simulink model "Revised_model_charging_station"  (Simulink 10.3)
settings: Solver=ode8  StartTime=0.0  StopTime=6  FixedStep=1e-04  RelTol=1e-3
undefined symbols (not defined in the file or in its folder): Acid, Lead
libraries: spsMosfetLib x14, spsDiodeLib x13, spsSeriesRLCBranchLib x12, simulink x9, spsCurrentMeasurementLib x8, pid_lib x7, spsBatteryLib x6, spsParallelRLCBranchLib x5, spsMeanLib x3, spsGroundLib x2, spsPWMGeneratorDCDCLib x2, spsVoltageMeasurementLib x2
settings Model: Creator=Devershi  LastModifiedBy=Aditya
settings Model: SuppressorTable=|
  | <?xml version="1.0" encoding="UTF-8" standalone="yes" ?>
  | <!DOCTYPE boost_serialization>
  | <boost_serialization signature="serialization::archive" version="17">
  | <DiagnosticSuppressor class_id="0" tracking_level="0" version="7">
  | 	<Table class_id="1" tracking_level="0" version="0">
  | 		<count>1</count>
  | 		<bucket_count>8</bucket_count>
  | 		<item_version>0</item_version>
  | 		<item class_id="2" tracking_level="0" version="0">
  | 			<first class_id="3" tracking_level="0" version="7">
  | 				<Source class_id="4" tracking_level="0" version="0">
  | 					<count>1</count>
  | 					<item_version>0</item_version>
  | 					<item>84:4</item>
  | 				</Source>
  | 			</first>
  | 			<second class_id="5" tracking_level="0" version="7">
  | 				<SuppressedData class_id="6" tracking_level="0" version="0">
  | 					<count>2</count>
  | 					<bucket_count>8</bucket_count>
  | 					<item_version>0</item_version>
  | 					<item class_id="7" tracking_level="0" version="0">
  | 						<first class_id="8" tracking_level="0" version="7">
  | 							<ID>SimulinkFixedPoint:util:Overflowoccurred</ID>
  | 							<Cause>
  | 								<Source>
  | 									<count>0</count>
  | 									<item_version>0</item_version>
  | 								</Source>
  | 							</Cause>
  | 						</first>
  | 						<second class_id="9" tracking_level="0" version="7">
  | 							<Comment></Comment>
  | 							<User></User>
  | 							<LastModified class_id="10" tracking_level="0" version="0">
  | 								<ptime_date class_id="11" tracking_level="0" version="0">
  | 									<date>20160608</date>
  | 								</ptime_date>
  | 								<ptime_time_duration class_id="12" tracking_level="0" version="1">
  | 									<is_special>0</is_special>
  | 									<time_duration_hours>15</time_duration_hours>
  | 									<time_duration_minutes>23</time_duration_minutes>
  | 									<time_duration_seconds>17</time_duration_seconds>
  | 									<time_duration_fractional_seconds>0</time_duration_fractional_seconds>
  | 								</ptime_time_duration>
  | 							</LastModified>
  | 							<SuppressionType>1</SuppressionType>
  | 						</second>
  | 					</item>
  | 					<item>
  | 						<first>
  | 							<ID>Simulink:DataType:WarningOverFlowDetected</ID>
  | 							<Cause>
  | 								<Source>
  | 									<count>0</count>
  | 									<item_version>0</item_version>
  | 								</Source>
  | 							</Cause>
  | 						</first>
  | 						<second>
  | 							<Comment></Comment>
  | 							<User></User>
  | 							<LastModified>
  | 								<ptime_date>
  | 									<date>20160608</date>
  | 								</ptime_date>
  | 								<ptime_time_duration>
  | 									<is_special>0</is_special>
  | 									<time_duration_hours>15</time_duration_hours>
  | 									<time_duration_minutes>23</time_duration_minutes>
  | 									<time_duration_seconds>17</time_duration_seconds>
  | 									<time_duration_fractional_seconds>0</time_duration_fractional_seconds>
  | 								</ptime_time_duration>
  | 							</LastModified>
  | 							<SuppressionType>1</SuppressionType>
  | 						</second>
  | 					</item>
  | 				</SuppressedData>
  | 			</second>
  | 		</item>
  | 	</Table>
  | </DiagnosticSuppressor>
  | 
  | </boost_serialization>
  | 
  | </boost_serialization>
settings SolverCC: AlgebraicLoopSolver=Auto
settings DataIOCC: SaveFormat=Dataset  SignalLoggingSaveFormat=Dataset  ReturnWorkspaceOutputs=on
settings OptimizationCC: ExpressionDepthLimit=128  LifeSpan=auto
settings DebuggingCC: UnderspecifiedInitializationDetection=Simplified  MergeDetectMultiDrivingBlocksExec=error  FcnCallInpInsideContextMsg=error  StateNameClashWarn=none  SFUnexpectedBacktrackingDiag=error  SFNoUnconditionalDefaultTransitionDiag=error  SFExecutionAtInitializationDiag=warning  SFMachineParentedDataDiag=error  ArithmeticOperatorsInVariantConditions=error
settings HardwareCC: ProdBitPerPointer=64  ProdBitPerSizeT=64  ProdBitPerPtrDiffT=64  ProdLargestAtomicFloat=Float  ProdIntDivRoundTo=Zero  ProdEndianess=LittleEndian  ProdWordSize=64  ProdHWDeviceType=Intel->x86-64 (Windows64)
settings ModelReferenceCC: PropagateSignalLabelsOutOfModel=on
settings SFSimCC: SimUseLocalCustomCode=on  CustomCodeUndefinedFunction=FilterOut
settings RTWCC: RTWUseLocalCustomCode=on
settings CodeAppCC: StateflowObjectComments=off
settings GRTTargetCC: TargetLangStandard=C99 (ISO)  CombineOutputUpdateFcns=on  GRTInterface=off
settings ConfigComp: CovMetricSettings=dwe  CovSaveCumulativeToWorkspaceVar=off  CovSaveSingleToWorkspaceVar=off  CovExternalEMLEnable=on

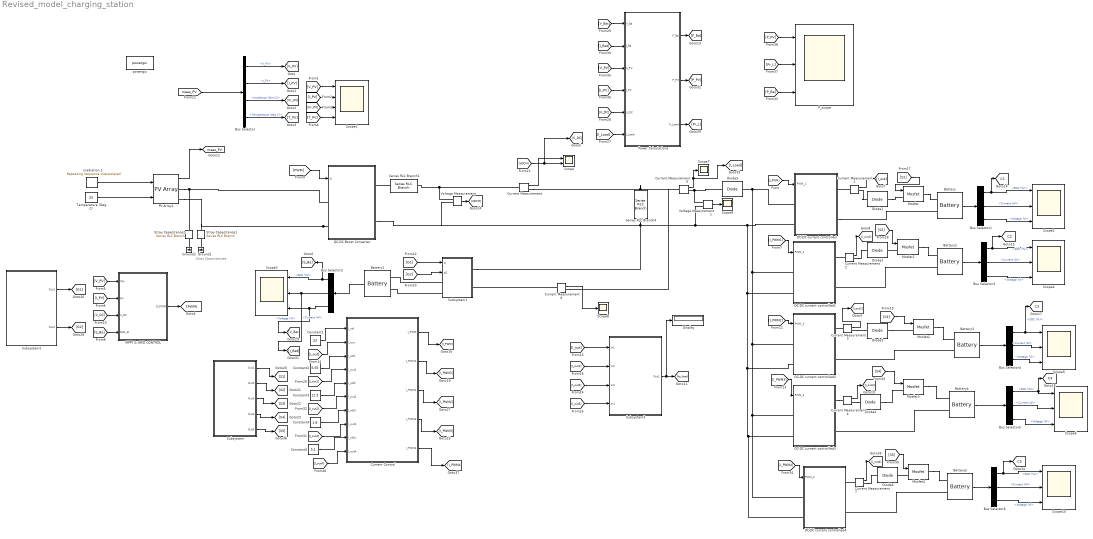
== system Revised_model_charging_station ==
  note: Stray
      | Capacitances
  Battery : spsBatteryLib/Battery  BatType=Lead-Acid  ShowTempParam=off  ThermalPreset=no  ShowAgeParam=off  NomV=72  NomQ=100  SOC=60  Batt_Tr=0.1  PresetModel=on  MaxQ=104.1667  MinV=54  FullV=78.3947  Dis_rate=20  R=0.0072  Normal_OP=31.0278  expZone="[73.3026     0.333333]"  current=[6.5 13 32.5]  Units=Time  Tci=20  NomT=20  T2=-30  MaxQ2=4.8  FullV2=7.1  Normal_OP2=5.655  expZone2="[6.58           1]"  Rca=0.6  ti=2000  Dp=0  Neq0=0  Tsim=1e6  Ta1=25  Qeol=5.4*0.9  Reol=0.013333*1.2  Char_age=[2.3478, 3]  Dis_age=[2.3478, 10]  N1=1500  N2=10500  N3=1000  N4=1400  Ta2=45  N5=950
  Battery1 : spsBatteryLib/Battery  BatType=Lead-Acid  ShowTempParam=off  ThermalPreset=no  ShowAgeParam=off  NomV=100  NomQ=150  SOC=65  Batt_Tr=0.1  PresetModel=on  MaxQ=156.25  MinV=75  FullV=108.8816  Dis_rate=30  R=0.0066667  Normal_OP=46.5417  expZone="[101.8092           0.5]"  current=[6.5 13 32.5]  Units=Time  Tci=20  NomT=20  T2=-30  MaxQ2=4.8  FullV2=7.1  Normal_OP2=5.655  expZone2="[6.58           1]"  Rca=0.6  ti=2000  Dp=0  Neq0=0  Tsim=1e6  Ta1=25  Qeol=5.4*0.9  Reol=0.013333*1.2  Char_age=[2.3478, 3]  Dis_age=[2.3478, 10]  N1=1500  N2=10500  N3=1000  N4=1400  Ta2=45  N5=950
  Battery2 : spsBatteryLib/Battery  BatType=Lead-Acid  ShowTempParam=off  ThermalPreset=no  ShowAgeParam=off  NomV=48  NomQ=37  SOC=30  Batt_Tr=0.1  PresetModel=on  MaxQ=38.5417  MinV=36  FullV=52.2632  Dis_rate=7.4  R=0.012973  Normal_OP=11.4803  expZone="[48.8684     0.123333]"  current=[6.5 13 32.5]  Units=Time  Tci=20  NomT=20  T2=-30  MaxQ2=4.8  FullV2=7.1  Normal_OP2=5.655  expZone2="[6.58           1]"  Rca=0.6  ti=2000  Dp=0  Neq0=0  Tsim=1e6  Ta1=25  Qeol=5.4*0.9  Reol=0.013333*1.2  Char_age=[2.3478, 3]  Dis_age=[2.3478, 10]  N1=1500  N2=10500  N3=1000  N4=1400  Ta2=45  N5=950
  Battery3 : spsBatteryLib/Battery  BatType=Lead-Acid  ShowTempParam=off  ThermalPreset=no  ShowAgeParam=off  NomV=48  NomQ=50  SOC=15  Batt_Tr=0.1  PresetModel=on  MaxQ=52.0833  MinV=36  FullV=52.2632  Dis_rate=10  R=0.0096  Normal_OP=15.5139  expZone="[48.8684     0.166667]"  current=[6.5 13 32.5]  Units=Time  Tci=20  NomT=20  T2=-30  MaxQ2=4.8  FullV2=7.1  Normal_OP2=5.655  expZone2="[6.58           1]"  Rca=0.6  ti=2000  Dp=0  Neq0=0  Tsim=1e6  Ta1=25  Qeol=5.4*0.9  Reol=0.013333*1.2  Char_age=[2.3478, 3]  Dis_age=[2.3478, 10]  N1=1500  N2=10500  N3=1000  N4=1400  Ta2=45  N5=950
  Battery4 : spsBatteryLib/Battery  BatType=Lead-Acid  ShowTempParam=off  ThermalPreset=no  ShowAgeParam=off  NomV=12  NomQ=18  SOC=90  Batt_Tr=0.1  PresetModel=on  MaxQ=18.75  MinV=9  FullV=13.0658  Dis_rate=3.6  R=0.0066667  Normal_OP=5.585  expZone="[12.2171         0.06]"  current=[6.5 13 32.5]  Units=Time  Tci=20  NomT=20  T2=-30  MaxQ2=4.8  FullV2=7.1  Normal_OP2=5.655  expZone2="[6.58           1]"  Rca=0.6  ti=2000  Dp=0  Neq0=0  Tsim=1e6  Ta1=25  Qeol=5.4*0.9  Reol=0.013333*1.2  Char_age=[2.3478, 3]  Dis_age=[2.3478, 10]  N1=1500  N2=10500  N3=1000  N4=1400  Ta2=45  N5=950
  Battery5 : spsBatteryLib/Battery  BatType=Lead-Acid  ShowTempParam=off  ThermalPreset=no  ShowAgeParam=off  NomV=48  NomQ=34  SOC=72  Batt_Tr=0.1  PresetModel=on  MaxQ=35.4167  MinV=36  FullV=52.2632  Dis_rate=6.8  R=0.014118  Normal_OP=10.5494  expZone="[48.8684     0.113333]"  current=[6.5 13 32.5]  Units=Time  Tci=20  NomT=20  T2=-30  MaxQ2=4.8  FullV2=7.1  Normal_OP2=5.655  expZone2="[6.58           1]"  Rca=0.6  ti=2000  Dp=0  Neq0=0  Tsim=1e6  Ta1=25  Qeol=5.4*0.9  Reol=0.013333*1.2  Char_age=[2.3478, 3]  Dis_age=[2.3478, 10]  N1=1500  N2=10500  N3=1000  N4=1400  Ta2=45  N5=950
  Bus Selector : BusSelector  OutputSignals=V_PV,I_PV,Irradiance (W/m2),Temperature (deg C)
  Bus Selector{1..6} (6 alike) : BusSelector  OutputSignals=SOC (%),Current (A),Voltage (V)
  Constant1 : Constant  Value=23
  Constant2 : Constant  Value=5.55
  Constant3 : Constant  Value=11.5
  Constant4 : Constant  Value=1.8
  Constant5 : Constant  Value=5.1
  Current Control : Subsystem
  Current Measurement{,1..7} (8 alike) : spsCurrentMeasurementLib/Current Measurement  PhasorSimulation=off  OutputType=Complex  PSBequivalent=0
  DC-DC Boost Converter : Subsystem
  DC-DC current controlled : Subsystem
  DC-DC current controlled1 : Subsystem
  DC-DC current controlled2 : Subsystem
  DC-DC current controlled3 : Subsystem
  DC-DC current controlled4 : Subsystem
  Diode{1..6} (6 alike) : spsDiodeLib/Diode  Ron=0.001  Lon=0  Vf=0.8  IC=0  UseSnubber=0  Rs=500  Cs=250e-9  Measurements=off
  Display : Display
  Ground1 : spsGroundLib/Ground  LConnTagsString=a
  Ground2 : spsGroundLib/Ground  LConnTagsString=a
  MPPT & GRID CONTROL : Subsystem
  Mosfet{,1..4} (5 alike) : spsMosfetLib/Mosfet  Ron=0.1  Lon=0  Rd=0.01  Vfd=0  IC=0  Rs=1e5  Cs=inf  Measurements=off
  PV Array1 : spsPVArrayLib/PV Array  Npar=8  Nser=8  PlotType=one module @ 25 deg.C & specified irradiances  S_vec="[ 1000 800 500  250 ]"  Temp_C_vec="[0 25 50  ]"  ModuleName=User-defined  PlotWhenSelected=on  Pm=204.7968  Ncell=60  Voc=22.46  Isc=11.65  Vm=18.72  Im=10.94  beta_Voc_pc=-0.3609  alpha_Isc_pc=0.102  beta_Voc=-0.081058  alpha_Isc=0.011883  IL=11.6575  I0=4.2837e-10  nI=0.60677  Rsh=131.4101  Rs=0.084786  RobustModel=off  RobustCellTemperature=25  BAL=on  Tc=Tc  Tfilter=5e-5
  P_scope : Scope  NumInputPorts=3
  Power Calculations : Subsystem
  Scope : Scope  NumInputPorts=2
  Scope1 : Scope  NumInputPorts=4
  Scope{2..6,10} (6 alike) : Scope  NumInputPorts=3
  Scope7 : Scope
  Scope8 : Scope
  Scope9 : Scope
  Series RLC Branch1 : spsSeriesRLCBranchLib/Series RLC Branch  LConnTagsString=__new0  RConnTagsString=__new0  BranchType=L  Resistance=1  Inductance=0.325e-3  SetiL0=off  InitialCurrent=0  Capacitance=15000e-6  Setx0=on  InitialVoltage=70  Measurements=None
  Series RLC Branch4 : spsSeriesRLCBranchLib/Series RLC Branch  LConnTagsString=__new0  RConnTagsString=__new0  BranchType=C  Resistance=1  Inductance=1e-3  SetiL0=off  InitialCurrent=0  Capacitance=15000e-6  Setx0=on  InitialVoltage=60  Measurements=None
  Stray Capacitance1 : spsSeriesRLCBranchLib/Series RLC Branch  LConnTagsString=__new0  RConnTagsString=__new0  BranchType=C  Resistance=1e-3  Inductance=1  SetiL0=off  InitialCurrent=0  Capacitance=4e-9  Setx0=off  InitialVoltage=0  Measurements=None
  Stray Capacitance2 : spsSeriesRLCBranchLib/Series RLC Branch  LConnTagsString=__new0  RConnTagsString=__new0  BranchType=C  Resistance=1e-3  Inductance=1  SetiL0=off  InitialCurrent=0  Capacitance=4e-9  Setx0=off  InitialVoltage=0  Measurements=None
  Subsystem : Subsystem
  Subsystem1 : Subsystem
  Subsystem2 : Subsystem
  Subsystem3 : Subsystem
  Temperature (Deg. C) : Constant  Value=25
  Voltage Measurement : spsVoltageMeasurementLib/Voltage Measurement  PhasorSimulation=off  OutputType=Complex  PSBequivalent=0
  Voltage Measurement1 : spsVoltageMeasurementLib/Voltage Measurement  PhasorSimulation=off  OutputType=Complex  PSBequivalent=0
  irradiation 2 : simulink/Sources/Repeating Sequence Interpolated  OutValues="[0 0  0 0 0 100 200 300 400 700 800 900 1000 975 900 800 700 400 300 200 0 0 0 0  ].'"  TimeValues=[0 0.25 0.50 0.75 1 1.25 1.50 1.75 2 2.25 2.75 3 3.25 3.50 3.75 4 4.25 4.5 4.75 5 5.25 5.5 5.75 6 ].'  LookUpMeth=Interpolation-Use End Values  tsamp=0.1  OutMin=[]  OutMax=[]  OutDataTypeStr=double  OutputDataTypeScalingMode=double  OutDataType=fixdt(0,8)  OutScaling=2^-10
  powergui : spspowerguiLib/powergui  Priority=1  SimulationMode=Discrete  SampleTime=1e-4  frequency=60  Iterations=50  frequencyindice=0  Pbase=100e6  ErrMax=1e-4  UnitsV=kV  UnitsW=MW  buscounter=0  FunctionMessages=off  echomessages=off  EnableUseOfTLC=off  CurrentSourceSwitches=off  DisableSnubberDevices=off  DisableRonSwitches=off  DisableVfSwitches=off  DisplayEquations=off  AutomaticDiscreteSolvers=off  SolverType=Tustin/Backward Euler (TBE)  Interpol=off  ExternalGateDelay=off  methode=off  Ts=100  x0status=blocks  SPID=on  SwTol=0  HookPort=off  NonlinearTolerance=1e-4  nMaxIteration=100  ContinueOnMaxIteration=off  RestoreLinks=warning  ResistiveCurrentMeasurement=off  Frange=[0:2:500]  Ylog=off  Xlog=on  ShowGrid=off  save=off  variable=ZData  structure=V_BATT  ZoomFFT=on  StartTime=0.604  cycles=7  DisplayStyle=1  fundamental=50  FreqAxis=off  MaxFrequency=200  frequencyindicesteady=1  RmsSteady=1  display=off
  tag scope: C1=global, C2=global, C3=global, C4=global, C5=global, No_load=global, meas_PV=global
  wires:
  Bus Selector5/2 -> Scope6/2  "<Current (A)>"
  Bus Selector5/3 -> Scope6/3  "<Voltage (V)>"
  Bus Selector5/1 -> [C4], Scope6/1  "<SOC (%)>"
  Battery2/1 -> Bus Selector3/1
  Bus Selector3/3 -> Scope4/3  "<Voltage (V)>"
  Bus Selector3/2 -> Scope4/2  "<Current (A)>"
  Battery/1 -> Bus Selector1/1
  Bus Selector1/3 -> Scope2/3  "<Voltage (V)>"
  Bus Selector/4 -> [T_PV]  "<Temperature (deg C)>"
  [meas_PV] -> Bus Selector/1
  [T_PV] -> Scope1/4
  Bus Selector/3 -> [Irr_PV]  "<Irradiance (W/m2)>"
  [I_PV] -> Scope1/2
  Bus Selector4/2 -> Scope5/2  "<Current (A)>"
  Bus Selector4/1 -> [C3], Scope5/1  "<SOC (%)>"
  Bus Selector/1 -> [V_PV]  "<V_PV>"
  Battery4/1 -> Bus Selector5/1
  Bus Selector/2 -> [I_PV]  "<I_PV>"
  [Irr_PV] -> Scope1/3
  Battery3/1 -> Bus Selector4/1
  PV Array1/1 -> [meas_PV]
  Temperature (Deg. C)/1 -> PV Array1/2
  Bus Selector3/1 -> [C2], Scope4/1  "<SOC (%)>"
  [PWM] -> DC-DC Boost Converter/1(D)
  [V_PV] -> Scope1/1
  Bus Selector1/1 -> [C1], Scope2/1  "<SOC (%)>"
  Bus Selector1/2 -> Scope2/2  "<Current (A)>"
  MPPT & GRID CONTROL/1(D_PWM) -> [PWM]
  Battery1/1 -> Bus Selector2/1
  [S_Ba] -> MPPT & GRID CONTROL/4(SOC_B)
  [V_DC] -> MPPT & GRID CONTROL/3(V_DC)
  [I_PV] -> MPPT & GRID CONTROL/2(Ipv)
  [V_PV] -> MPPT & GRID CONTROL/1(Vpv)
  Bus Selector2/1 -> [S_Ba], Scope3/1  "<SOC (%)>"
  Bus Selector2/3 -> [V_Bat], Scope3/3  "<Voltage (V)>"
  Bus Selector2/2 -> [I_Bat], Scope3/2  "<Current (A)>"
  Bus Selector4/3 -> Scope5/3  "<Voltage (V)>"
  [I_out] -> Current Control/2(I_out)
  Constant1/1 -> Current Control/1(I_ref)
  Current Control/1(I_PWM) -> [I_PWM]
  Constant2/1 -> Current Control/3(I_ref1)
  Current Control/2(I_PWM1) -> [I_PWM1]
  [I_out3] -> Current Control/8(I_out3)
  [I_out2] -> Current Control/6(I_out2)
  Current Control/3(I_PWM2) -> [I_PWM2]
  Constant4/1 -> Current Control/7(I_ref3)
  Current Control/4(I_PWM3) -> [I_PWM3]
  Constant3/1 -> Current Control/5(I_ref2)
  [I_out1] -> Current Control/4(I_out1)
  [I_PWM] -> DC-DC current controlled/1(PWM_1)
  Current Measurement1/1 -> [I_out]
  Current Measurement2/1 -> [I_out1]
  Current Measurement3/1 -> [I_out2]
  Current Measurement4/1 -> [I_out3]
  [I_PWM1] -> DC-DC current controlled1/1(PWM_2)
  [I_PWM2] -> DC-DC current controlled2/1(PWM_3)
  [I_PWM3] -> DC-DC current controlled3/1(PWM_4)
  irradiation 2/1 -> PV Array1/1
  Subsystem/1(Out1) -> [S1]
  Subsystem/2(Out2) -> [S2]
  Subsystem/3(Out3) -> [S3]
  Subsystem/4(Out4) -> [S4]
  [S1] -> Mosfet/1
  [S2] -> Mosfet1/1
  [S3] -> Mosfet2/1
  [S4] -> Mosfet3/1
  [G1] -> Subsystem1/1(g)
  [G2] -> Subsystem1/2(g1)
  Subsystem2/1(Out1) -> [G1]
  Subsystem2/2(Out2) -> [G2]
  [VDCM] -> [V_DC], Scope/2
  Current Measurement/1 -> Scope/1
  Voltage Measurement/1 -> [VDCM]
  [I_out] -> Subsystem3/1(In1)
  [I_out1] -> Subsystem3/2(In2)
  [I_out2] -> Subsystem3/3(In3)
  [I_out3] -> Subsystem3/4(In4)
  Subsystem3/1(Out1) -> Display/1, [No_load]
  Current Measurement6/1 -> Scope8/1
  Current Measurement5/1 -> [I_Load], Scope7/1
  Voltage Measurement1/1 -> Scope9/1
  Power Calculations/1(P_Ba) -> [P_Ba]
  Power Calculations/3(P_Load) -> [Pr_L]
  [V_Bat] -> Power Calculations/1(V_Ba)
  [I_Bat] -> Power Calculations/2(I_Ba)
  [I_Load] -> Power Calculations/6(I_Load)
  [V_DC] -> Power Calculations/5(V_DC)
  Power Calculations/2(P_PV) -> [P_PV]
  [I_PV] -> Power Calculations/4(I_PV)
  [V_PV] -> Power Calculations/3(V_PV)
  [Pr_L] -> P_scope/2
  [P_PV] -> P_scope/1
  [P_Ba] -> P_scope/3
  [I_PWM4] -> DC-DC current controlled4/1(PWM_2)
  Current Measurement7/1 -> [I_out4]
  Bus Selector6/1 -> Scope10/1, [C5]  "<SOC (%)>"
  Bus Selector6/2 -> Scope10/2  "<Current (A)>"
  Bus Selector6/3 -> Scope10/3  "<Voltage (V)>"
  Battery5/1 -> Bus Selector6/1
  [S5] -> Mosfet4/1
  Subsystem/5(Out5) -> [S5]
  Constant5/1 -> Current Control/9(I_ref4)
  [I_out4] -> Current Control/10(I_out4)
  Current Control/5(I_PWM4) -> [I_PWM4]
  connections:
  Stray Capacitance2/LConn1 -- DC-DC Boost Converter/LConn1 -- PV Array1/RConn1
  DC-DC Boost Converter/LConn2 -- PV Array1/RConn2 -- Stray Capacitance1/LConn1
  Ground1/LConn1 -- Stray Capacitance1/RConn1
  Ground2/LConn1 -- Stray Capacitance2/RConn1
  Current Measurement1/LConn1 -- DC-DC current controlled/RConn1
  Diode1/LConn1 -- Current Measurement1/RConn1
  DC-DC current controlled3/RConn1 -- Current Measurement4/LConn1
  Current Measurement4/RConn1 -- Diode4/LConn1
  Current Measurement3/LConn1 -- DC-DC current controlled2/RConn1
  Current Measurement3/RConn1 -- Diode3/LConn1
  Current Measurement2/LConn1 -- DC-DC current controlled1/RConn1
  Current Measurement2/RConn1 -- Diode2/LConn1
  DC-DC current controlled3/LConn1 -- DC-DC current controlled4/LConn1 -- DC-DC current controlled2/LConn1 -- DC-DC current controlled1/LConn1 -- DC-DC current controlled/LConn1 -- Diode5/RConn1
  Diode1/RConn1 -- Mosfet/LConn1
  Diode4/RConn1 -- Mosfet3/LConn1
  Diode3/RConn1 -- Mosfet2/LConn1
  Subsystem1/LConn1 -- Battery1/LConn1
  Subsystem1/LConn2 -- Battery1/LConn2
  Mosfet1/LConn1 -- Diode2/RConn1
  DC-DC current controlled3/LConn2 -- DC-DC current controlled4/LConn2 -- DC-DC current controlled2/LConn2 -- DC-DC current controlled1/LConn2 -- Voltage Measurement1/LConn2 -- Subsystem1/RConn1 -- DC-DC Boost Converter/RConn2 -- Voltage Measurement/LConn2 -- Series RLC Branch4/RConn1 -- DC-DC current controlled/LConn2
  Voltage Measurement/LConn1 -- Current Measurement/LConn1 -- Series RLC Branch1/LConn1
  Series RLC Branch4/LConn1 -- Current Measurement6/RConn1 -- Current Measurement5/LConn1 -- Current Measurement/RConn1
  Series RLC Branch1/RConn1 -- DC-DC Boost Converter/RConn1
  Current Measurement5/RConn1 -- Voltage Measurement1/LConn1 -- Diode5/LConn1
  Mosfet/RConn1 -- Battery/LConn1
  DC-DC current controlled/RConn2 -- Battery/LConn2
  Mosfet1/RConn1 -- Battery2/LConn1
  Battery2/LConn2 -- DC-DC current controlled1/RConn2
  Mosfet2/RConn1 -- Battery3/LConn1
  Battery3/LConn2 -- DC-DC current controlled2/RConn2
  Mosfet3/RConn1 -- Battery4/LConn1
  Battery4/LConn2 -- DC-DC current controlled3/RConn2
  Current Measurement6/LConn1 -- Subsystem1/RConn2
  Battery5/LConn2 -- DC-DC current controlled4/RConn2
  Mosfet4/RConn1 -- Battery5/LConn1
  Current Measurement7/RConn1 -- Diode6/LConn1
  Current Measurement7/LConn1 -- DC-DC current controlled4/RConn1
  Mosfet4/LConn1 -- Diode6/RConn1

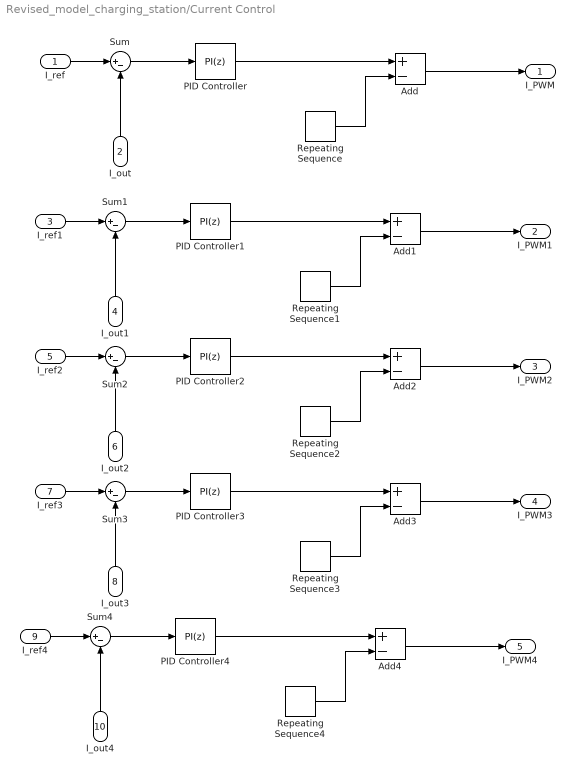
== system Revised_model_charging_station/Current Control ==
  I_ref : Inport
  I_out : Inport  Port=2
  I_ref1 : Inport  Port=3
  I_out1 : Inport  Port=4
  I_ref2 : Inport  Port=5
  I_out2 : Inport  Port=6
  I_ref3 : Inport  Port=7
  I_out3 : Inport  Port=8
  I_ref4 : Inport  Port=9
  I_out4 : Inport  Port=10
  Add{,1..4} (5 alike) : Sum  Inputs=+-
  PID Controller{,1..4} (5 alike) : pid_lib/PID Controller  Controller=PI  Form=Parallel  TimeDomain=Discrete-time  UseExternalTs=off  SampleTime=-1  IntegratorMethod=Forward Euler  FilterMethod=Forward Euler  ControllerParametersSource=internal  P=0.4928  I=0.93  D=0  UseFilter=on  N=100  TunerSelectOption=Transfer Function Based (PID Tuner App)  InitialConditionSource=internal  InitialConditionForIntegrator=0  InitialConditionForFilter=0  DifferentiatorICPrevScaledInput=0  ExternalReset=none  TrackingMode=off  Kt=1  LimitOutput=off  SatLimitsSource=internal  UpperSaturationLimit=inf  LowerSaturationLimit=-inf  LinearizeAsGain=on  AntiWindupMode=none  Kb=1  POutMin=[]  POutMax=[]  IOutMin=[]  IOutMax=[]  DOutMin=[]  DOutMax=[]  NOutMin=[]  NOutMax=[]  SumOutMin=[]  SumOutMax=[]  SaturationOutMin=[]  SaturationOutMax=[]  PParamMin=[]  PParamMax=[]  IParamMin=[]  IParamMax=[]  DParamMin=[]  DParamMax=[]  NParamMin=[]  NParamMax=[]  KbParamMin=[]  KbParamMax=[]  KtParamMin=[]  KtParamMax=[]  KbOutMin=[]  KbOutMax=[]  KtOutMin=[]  KtOutMax=[]  IntegratorOutMin=[]  IntegratorOutMax=[]  FilterOutMin=[]  FilterOutMax=[]  SumI1OutMin=[]  SumI1OutMax=[]  SumI2OutMin=[]  SumI2OutMax=[]  SumI3OutMin=[]  SumI3OutMax=[]  SumI4OutMin=[]  SumI4OutMax=[]  SumDOutMin=[]  SumDOutMax=[]  DifferentiatorOutMin=[]  DifferentiatorOutMax=[]  FilterDiffOutCoefMin=[]  FilterDiffOutCoefMax=[]  ReciprocalOutMin=[]  ReciprocalOutMax=[]  SumDenOutMin=[]  SumDenOutMax=[]  SumNumOutMin=[]  SumNumOutMax=[]  DivideOutMin=[]  DivideOutMax=[]  UdiffTsProdOutMin=[]  UdiffTsProdOutMax=[]  NTsProdOutMin=[]  NTsProdOutMax=[]  UintegralTsProdOutMin=[]  UintegralTsProdOutMax=[]  UngainTsProdOutMin=[]  UngainTsProdOutMax=[]  IntegratorContinuousStateAttributes=''  IntegratorStateMustResolveToSignalObject=off  IntegratorRTWStateStorageClass=Auto  FilterContinuousStateAttributes=''  FilterStateMustResolveToSignalObject=off  FilterRTWStateStorageClass=Auto  ParallelPVariant=InternalParameters  IdealPVariant=Disabled  IVariant=InternalParameters  DVariant=Disabled  IntegratorVariant=Discrete  SatVariant=Disabled  AWVariant=Passthrough  PCopyVariant=Disabled  TRVariant=Disabled  FdbkBlocksVariant=Forward  IdealPFdbkVariant=Disabled  SatFdbkVariant=Disabled  DerivativeFilterVariant=Disabled  NVariant=Disabled  NCopyVariant=Disabled_SignalSpec  FilterICVariant=Disabled  IntegratorICVariant=InternalICs  ExternalResetVariant=Disabled  TRSumVariant=Passthrough  SumFdbkVariant=Disabled  SumVariant=Sum_PI  TsampFilterVariant=InternalTs  TsampNgainVariant=Passthrough  TsampIntegralVariant=Passthrough  ExternalSaturationOutDataTypeStr=Inherit: Same as second input
  Repeating Sequence{,1..4} (5 alike) : simulink/Sources/Repeating Sequence  rep_seq_t=[0 0.25/5000 0.5/5000 0.75/5000 1/5000]  rep_seq_y=[0 -1 0 1 0]
  Sum{,1..4} (5 alike) : Sum  Inputs=|+-
  I_PWM : Outport
  I_PWM1 : Outport  Port=2
  I_PWM2 : Outport  Port=3
  I_PWM3 : Outport  Port=4
  I_PWM4 : Outport  Port=5
  wires:
  Sum/1 -> PID Controller/1
  PID Controller/1 -> Add/1
  Repeating Sequence/1 -> Add/2
  I_out/1 -> Sum/2
  Add/1 -> I_PWM/1
  I_ref/1 -> Sum/1
  I_ref1/1 -> Sum1/1
  Add1/1 -> I_PWM1/1
  I_out1/1 -> Sum1/2
  Repeating Sequence1/1 -> Add1/2
  PID Controller1/1 -> Add1/1
  Sum1/1 -> PID Controller1/1
  Sum2/1 -> PID Controller2/1
  PID Controller2/1 -> Add2/1
  Repeating Sequence2/1 -> Add2/2
  I_out2/1 -> Sum2/2
  Add2/1 -> I_PWM2/1
  I_ref2/1 -> Sum2/1
  I_ref3/1 -> Sum3/1
  Add3/1 -> I_PWM3/1
  I_out3/1 -> Sum3/2
  Repeating Sequence3/1 -> Add3/2
  PID Controller3/1 -> Add3/1
  Sum3/1 -> PID Controller3/1
  Sum4/1 -> PID Controller4/1
  PID Controller4/1 -> Add4/1
  Repeating Sequence4/1 -> Add4/2
  I_out4/1 -> Sum4/2
  Add4/1 -> I_PWM4/1
  I_ref4/1 -> Sum4/1

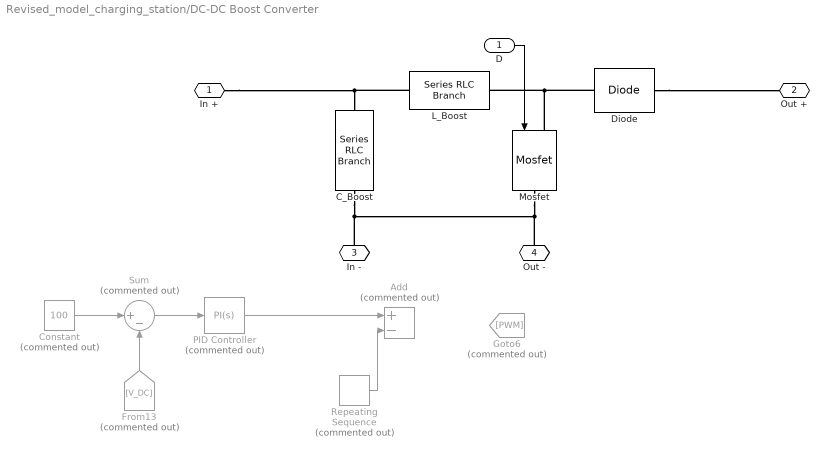
== system Revised_model_charging_station/DC-DC Boost Converter ==
  D : Inport
  Add : Sum  Commented=on  Inputs=+-
  C_Boost : spsSeriesRLCBranchLib/Series RLC Branch  LConnTagsString=__new0  RConnTagsString=__new0  BranchType=C  Resistance=0.01  Inductance=1e-3  SetiL0=off  InitialCurrent=0  Capacitance=15000e-6  Setx0=off  InitialVoltage=0  Measurements=None
  Constant : Constant  Commented=on  Value=100
  Diode : spsDiodeLib/Diode  Ron=0.001  Lon=0  Vf=0.8  IC=0  UseSnubber=0  Rs=500  Cs=250e-9  Measurements=off
  From13 : From  Commented=on  GotoTag=V_DC  TagVisibility=global
  Goto6 : Goto  Commented=on  GotoTag=PWM
  L_Boost : spsSeriesRLCBranchLib/Series RLC Branch  LConnTagsString=__new0  RConnTagsString=__new0  BranchType=RL  Resistance=0.05  Inductance=0.325e-3  SetiL0=off  InitialCurrent=0  Capacitance=1e-6  Setx0=off  InitialVoltage=0  Measurements=None
  Mosfet : spsMosfetLib/Mosfet  Ron=0.1  Lon=0  Rd=0.01  Vfd=0  IC=0  Rs=1e5  Cs=inf  Measurements=off
  PID Controller : pid_lib/PID Controller  Commented=on  Controller=PI  Form=Parallel  TimeDomain=Continuous-time  UseExternalTs=off  SampleTime=-1  IntegratorMethod=Forward Euler  FilterMethod=Forward Euler  ControllerParametersSource=internal  P=0.00311454767329859  I=0.000230615968798365  D=0  UseFilter=on  N=100  TunerSelectOption=Transfer Function Based (PID Tuner App)  InitialConditionSource=internal  InitialConditionForIntegrator=0  InitialConditionForFilter=0  DifferentiatorICPrevScaledInput=0  ExternalReset=none  TrackingMode=off  Kt=1  LimitOutput=off  SatLimitsSource=internal  UpperSaturationLimit=inf  LowerSaturationLimit=-inf  LinearizeAsGain=on  AntiWindupMode=none  Kb=1  POutMin=[]  POutMax=[]  IOutMin=[]  IOutMax=[]  DOutMin=[]  DOutMax=[]  NOutMin=[]  NOutMax=[]  SumOutMin=[]  SumOutMax=[]  SaturationOutMin=[]  SaturationOutMax=[]  PParamMin=[]  PParamMax=[]  IParamMin=[]  IParamMax=[]  DParamMin=[]  DParamMax=[]  NParamMin=[]  NParamMax=[]  KbParamMin=[]  KbParamMax=[]  KtParamMin=[]  KtParamMax=[]  KbOutMin=[]  KbOutMax=[]  KtOutMin=[]  KtOutMax=[]  IntegratorOutMin=[]  IntegratorOutMax=[]  FilterOutMin=[]  FilterOutMax=[]  SumI1OutMin=[]  SumI1OutMax=[]  SumI2OutMin=[]  SumI2OutMax=[]  SumI3OutMin=[]  SumI3OutMax=[]  SumI4OutMin=[]  SumI4OutMax=[]  SumDOutMin=[]  SumDOutMax=[]  DifferentiatorOutMin=[]  DifferentiatorOutMax=[]  FilterDiffOutCoefMin=[]  FilterDiffOutCoefMax=[]  ReciprocalOutMin=[]  ReciprocalOutMax=[]  SumDenOutMin=[]  SumDenOutMax=[]  SumNumOutMin=[]  SumNumOutMax=[]  DivideOutMin=[]  DivideOutMax=[]  UdiffTsProdOutMin=[]  UdiffTsProdOutMax=[]  NTsProdOutMin=[]  NTsProdOutMax=[]  UintegralTsProdOutMin=[]  UintegralTsProdOutMax=[]  UngainTsProdOutMin=[]  UngainTsProdOutMax=[]  IntegratorContinuousStateAttributes=''  IntegratorStateMustResolveToSignalObject=off  IntegratorRTWStateStorageClass=Auto  FilterContinuousStateAttributes=''  FilterStateMustResolveToSignalObject=off  FilterRTWStateStorageClass=Auto  ParallelPVariant=InternalParameters  IdealPVariant=Disabled  IVariant=InternalParameters  DVariant=Disabled  IntegratorVariant=Continuous  SatVariant=Disabled  AWVariant=Passthrough  PCopyVariant=Disabled  TRVariant=Disabled  FdbkBlocksVariant=Forward  IdealPFdbkVariant=Disabled  SatFdbkVariant=Disabled  DerivativeFilterVariant=Disabled  NVariant=Disabled  NCopyVariant=Disabled_SignalSpec  FilterICVariant=Disabled  IntegratorICVariant=InternalICs  ExternalResetVariant=Disabled  TRSumVariant=Passthrough  SumFdbkVariant=Disabled  SumVariant=Sum_PI  TsampFilterVariant=InternalTs  TsampNgainVariant=Passthrough  TsampIntegralVariant=Passthrough  ExternalSaturationOutDataTypeStr=Inherit: Same as second input
  Repeating Sequence : simulink/Sources/Repeating Sequence  Commented=on  rep_seq_t=[0 0.25/5000 0.5/5000 0.75/5000 1/5000]  rep_seq_y=[0 -1 0 1 0]
  Sum : Sum  Commented=on  Inputs=|+-
  In + : PMIOPort  Side=Left
  Out + : PMIOPort  Port=2  Side=Right
  In - : PMIOPort  Port=3  Side=Left
  Out - : PMIOPort  Port=4  Side=Right
  wires:
  Constant/1 -> Sum/1
  From13/1 -> Sum/2
  Sum/1 -> PID Controller/1
  PID Controller/1 -> Add/1
  Repeating Sequence/1 -> Add/2
  D/1 -> Mosfet/1
  connections:
  Mosfet/LConn1 -- Diode/LConn1 -- L_Boost/RConn1
  Diode/RConn1 -- Out +/RConn1
  L_Boost/LConn1 -- In +/RConn1 -- C_Boost/LConn1
  C_Boost/RConn1 -- In -/RConn1 -- Mosfet/RConn1 -- Out -/RConn1

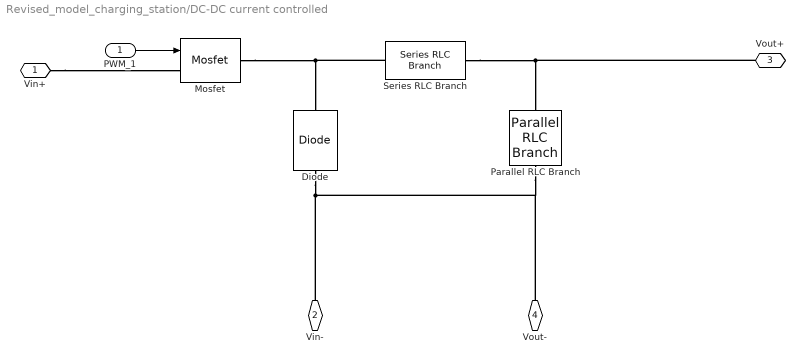
== system Revised_model_charging_station/DC-DC current controlled ==
  PWM_1 : Inport
  Diode : spsDiodeLib/Diode  Ron=0.001  Lon=0  Vf=0.8  IC=0  UseSnubber=0  Rs=500  Cs=250e-9  Measurements=off
  Mosfet : spsMosfetLib/Mosfet  Ron=0.1  Lon=0  Rd=0.01  Vfd=0  IC=0  Rs=1e5  Cs=inf  Measurements=off
  Parallel RLC Branch : spsParallelRLCBranchLib/Parallel RLC Branch  LConnTagsString=a  RConnTagsString=__new0  BranchType=C  Resistance=1  Inductance=1e-3  SetiL0=off  InitialCurrent=0  Capacitance=200e-6  Setx0=off  InitialVoltage=0  Measurements=None
  Series RLC Branch : spsSeriesRLCBranchLib/Series RLC Branch  LConnTagsString=__new0  RConnTagsString=__new0  BranchType=L  Resistance=10  Inductance=100e-3  SetiL0=off  InitialCurrent=0  Capacitance=1e-6  Setx0=off  InitialVoltage=0  Measurements=None
  Vin+ : PMIOPort  Side=Left
  Vin- : PMIOPort  Port=2  Side=Left
  Vout+ : PMIOPort  Port=3  Side=Right
  Vout- : PMIOPort  Port=4  Side=Right
  wires:
  PWM_1/1 -> Mosfet/1
  connections:
  Mosfet/RConn1 -- Diode/RConn1 -- Series RLC Branch/LConn1
  Vin-/RConn1 -- Vout-/RConn1 -- Parallel RLC Branch/RConn1 -- Diode/LConn1
  Vout+/RConn1 -- Series RLC Branch/RConn1 -- Parallel RLC Branch/LConn1
  Vin+/RConn1 -- Mosfet/LConn1

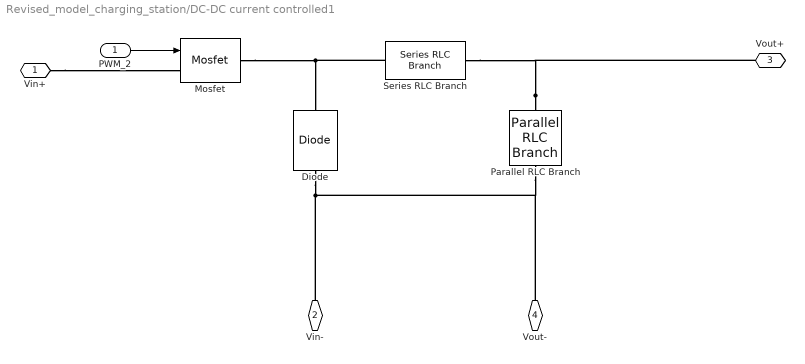
== system Revised_model_charging_station/DC-DC current controlled1 ==
  PWM_2 : Inport
  Diode : spsDiodeLib/Diode  Ron=0.001  Lon=0  Vf=0.8  IC=0  UseSnubber=0  Rs=500  Cs=250e-9  Measurements=off
  Mosfet : spsMosfetLib/Mosfet  Ron=0.1  Lon=0  Rd=0.01  Vfd=0  IC=0  Rs=1e5  Cs=inf  Measurements=off
  Parallel RLC Branch : spsParallelRLCBranchLib/Parallel RLC Branch  LConnTagsString=a  RConnTagsString=__new0  BranchType=C  Resistance=1  Inductance=1e-3  SetiL0=off  InitialCurrent=0  Capacitance=200e-6  Setx0=off  InitialVoltage=0  Measurements=None
  Series RLC Branch : spsSeriesRLCBranchLib/Series RLC Branch  LConnTagsString=__new0  RConnTagsString=__new0  BranchType=L  Resistance=10  Inductance=100e-3  SetiL0=off  InitialCurrent=0  Capacitance=1e-6  Setx0=off  InitialVoltage=0  Measurements=None
  Vin+ : PMIOPort  Side=Left
  Vin- : PMIOPort  Port=2  Side=Left
  Vout+ : PMIOPort  Port=3  Side=Right
  Vout- : PMIOPort  Port=4  Side=Right
  wires:
  PWM_2/1 -> Mosfet/1
  connections:
  Vin+/RConn1 -- Mosfet/LConn1
  Parallel RLC Branch/LConn1 -- Series RLC Branch/RConn1 -- Vout+/RConn1
  Diode/LConn1 -- Parallel RLC Branch/RConn1 -- Vout-/RConn1 -- Vin-/RConn1
  Series RLC Branch/LConn1 -- Diode/RConn1 -- Mosfet/RConn1

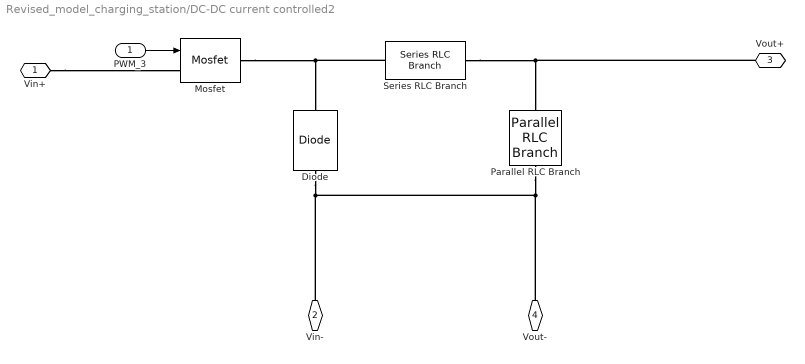
== system Revised_model_charging_station/DC-DC current controlled2 ==
  PWM_3 : Inport
  Diode : spsDiodeLib/Diode  Ron=0.001  Lon=0  Vf=0.8  IC=0  UseSnubber=0  Rs=500  Cs=250e-9  Measurements=off
  Mosfet : spsMosfetLib/Mosfet  Ron=0.1  Lon=0  Rd=0.01  Vfd=0  IC=0  Rs=1e5  Cs=inf  Measurements=off
  Parallel RLC Branch : spsParallelRLCBranchLib/Parallel RLC Branch  LConnTagsString=a  RConnTagsString=__new0  BranchType=C  Resistance=1  Inductance=1e-3  SetiL0=off  InitialCurrent=0  Capacitance=200e-6  Setx0=off  InitialVoltage=0  Measurements=None
  Series RLC Branch : spsSeriesRLCBranchLib/Series RLC Branch  LConnTagsString=__new0  RConnTagsString=__new0  BranchType=L  Resistance=10  Inductance=100e-3  SetiL0=off  InitialCurrent=0  Capacitance=1e-6  Setx0=off  InitialVoltage=0  Measurements=None
  Vin+ : PMIOPort  Side=Left
  Vin- : PMIOPort  Port=2  Side=Left
  Vout+ : PMIOPort  Port=3  Side=Right
  Vout- : PMIOPort  Port=4  Side=Right
  wires:
  PWM_3/1 -> Mosfet/1
  connections:
  Mosfet/RConn1 -- Diode/RConn1 -- Series RLC Branch/LConn1
  Vin-/RConn1 -- Vout-/RConn1 -- Parallel RLC Branch/RConn1 -- Diode/LConn1
  Vout+/RConn1 -- Series RLC Branch/RConn1 -- Parallel RLC Branch/LConn1
  Vin+/RConn1 -- Mosfet/LConn1

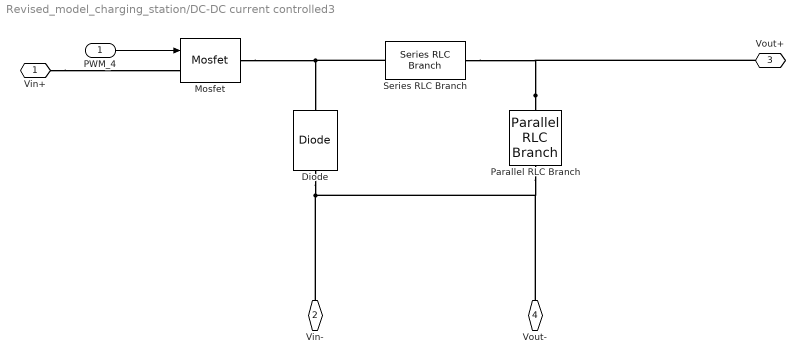
== system Revised_model_charging_station/DC-DC current controlled3 ==
  PWM_4 : Inport
  Diode : spsDiodeLib/Diode  Ron=0.001  Lon=0  Vf=0.8  IC=0  UseSnubber=0  Rs=500  Cs=250e-9  Measurements=off
  Mosfet : spsMosfetLib/Mosfet  Ron=0.1  Lon=0  Rd=0.01  Vfd=0  IC=0  Rs=1e5  Cs=inf  Measurements=off
  Parallel RLC Branch : spsParallelRLCBranchLib/Parallel RLC Branch  LConnTagsString=a  RConnTagsString=__new0  BranchType=C  Resistance=1  Inductance=1e-3  SetiL0=off  InitialCurrent=0  Capacitance=200e-6  Setx0=off  InitialVoltage=0  Measurements=None
  Series RLC Branch : spsSeriesRLCBranchLib/Series RLC Branch  LConnTagsString=__new0  RConnTagsString=__new0  BranchType=L  Resistance=10  Inductance=100e-3  SetiL0=off  InitialCurrent=0  Capacitance=1e-6  Setx0=off  InitialVoltage=0  Measurements=None
  Vin+ : PMIOPort  Side=Left
  Vin- : PMIOPort  Port=2  Side=Left
  Vout+ : PMIOPort  Port=3  Side=Right
  Vout- : PMIOPort  Port=4  Side=Right
  wires:
  PWM_4/1 -> Mosfet/1
  connections:
  Vin+/RConn1 -- Mosfet/LConn1
  Parallel RLC Branch/LConn1 -- Series RLC Branch/RConn1 -- Vout+/RConn1
  Diode/LConn1 -- Parallel RLC Branch/RConn1 -- Vout-/RConn1 -- Vin-/RConn1
  Series RLC Branch/LConn1 -- Diode/RConn1 -- Mosfet/RConn1

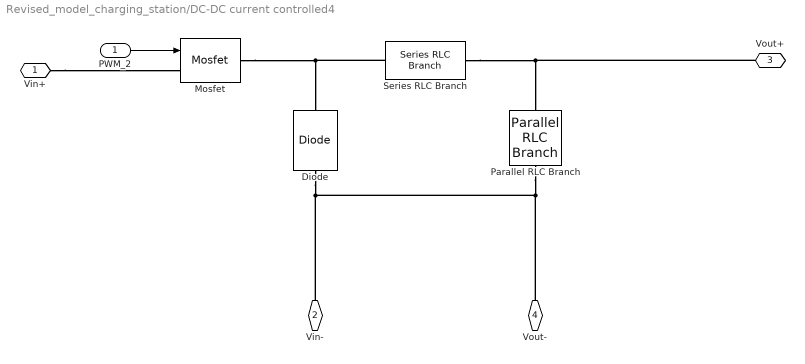
== system Revised_model_charging_station/DC-DC current controlled4 ==
  PWM_2 : Inport
  Diode : spsDiodeLib/Diode  Ron=0.001  Lon=0  Vf=0.8  IC=0  UseSnubber=0  Rs=500  Cs=250e-9  Measurements=off
  Mosfet : spsMosfetLib/Mosfet  Ron=0.1  Lon=0  Rd=0.01  Vfd=0  IC=0  Rs=1e5  Cs=inf  Measurements=off
  Parallel RLC Branch : spsParallelRLCBranchLib/Parallel RLC Branch  LConnTagsString=a  RConnTagsString=__new0  BranchType=C  Resistance=1  Inductance=1e-3  SetiL0=off  InitialCurrent=0  Capacitance=200e-6  Setx0=off  InitialVoltage=0  Measurements=None
  Series RLC Branch : spsSeriesRLCBranchLib/Series RLC Branch  LConnTagsString=__new0  RConnTagsString=__new0  BranchType=L  Resistance=10  Inductance=100e-3  SetiL0=off  InitialCurrent=0  Capacitance=1e-6  Setx0=off  InitialVoltage=0  Measurements=None
  Vin+ : PMIOPort  Side=Left
  Vin- : PMIOPort  Port=2  Side=Left
  Vout+ : PMIOPort  Port=3  Side=Right
  Vout- : PMIOPort  Port=4  Side=Right
  wires:
  PWM_2/1 -> Mosfet/1
  connections:
  Mosfet/RConn1 -- Diode/RConn1 -- Series RLC Branch/LConn1
  Vin-/RConn1 -- Vout-/RConn1 -- Parallel RLC Branch/RConn1 -- Diode/LConn1
  Vout+/RConn1 -- Series RLC Branch/RConn1 -- Parallel RLC Branch/LConn1
  Vin+/RConn1 -- Mosfet/LConn1

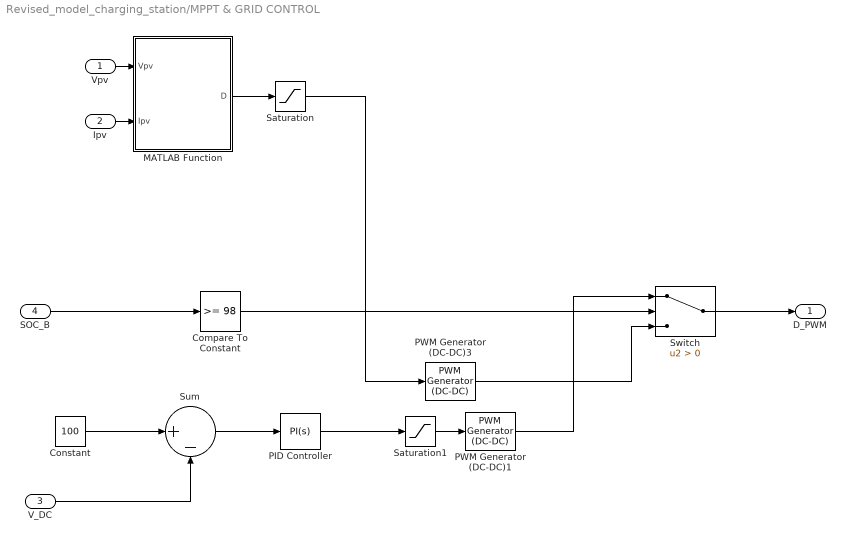
== system Revised_model_charging_station/MPPT & GRID CONTROL ==
  Vpv : Inport
  Ipv : Inport  Port=2
  V_DC : Inport  Port=3
  SOC_B : Inport  Port=4
  Compare To Constant : simulink/Logic and Bit Operations/Compare To Constant  relop=>=  const=98  OutDataTypeStr=boolean
  Constant : Constant  Value=100
  MATLAB Function : MATLAB Function  TreatAsAtomicUnit=on
  PID Controller : pid_lib/PID Controller  Controller=PI  Form=Parallel  TimeDomain=Continuous-time  UseExternalTs=off  SampleTime=-1  IntegratorMethod=Forward Euler  FilterMethod=Forward Euler  ControllerParametersSource=internal  P=0.1  I=0.1  D=0  UseFilter=on  N=100  TunerSelectOption=Transfer Function Based (PID Tuner App)  InitialConditionSource=internal  InitialConditionForIntegrator=0  InitialConditionForFilter=0  DifferentiatorICPrevScaledInput=0  ExternalReset=none  TrackingMode=off  Kt=1  LimitOutput=off  SatLimitsSource=internal  UpperSaturationLimit=inf  LowerSaturationLimit=-inf  LinearizeAsGain=on  AntiWindupMode=none  Kb=1  POutMin=[]  POutMax=[]  IOutMin=[]  IOutMax=[]  DOutMin=[]  DOutMax=[]  NOutMin=[]  NOutMax=[]  SumOutMin=[]  SumOutMax=[]  SaturationOutMin=[]  SaturationOutMax=[]  PParamMin=[]  PParamMax=[]  IParamMin=[]  IParamMax=[]  DParamMin=[]  DParamMax=[]  NParamMin=[]  NParamMax=[]  KbParamMin=[]  KbParamMax=[]  KtParamMin=[]  KtParamMax=[]  KbOutMin=[]  KbOutMax=[]  KtOutMin=[]  KtOutMax=[]  IntegratorOutMin=[]  IntegratorOutMax=[]  FilterOutMin=[]  FilterOutMax=[]  SumI1OutMin=[]  SumI1OutMax=[]  SumI2OutMin=[]  SumI2OutMax=[]  SumI3OutMin=[]  SumI3OutMax=[]  SumI4OutMin=[]  SumI4OutMax=[]  SumDOutMin=[]  SumDOutMax=[]  DifferentiatorOutMin=[]  DifferentiatorOutMax=[]  FilterDiffOutCoefMin=[]  FilterDiffOutCoefMax=[]  ReciprocalOutMin=[]  ReciprocalOutMax=[]  SumDenOutMin=[]  SumDenOutMax=[]  SumNumOutMin=[]  SumNumOutMax=[]  DivideOutMin=[]  DivideOutMax=[]  UdiffTsProdOutMin=[]  UdiffTsProdOutMax=[]  NTsProdOutMin=[]  NTsProdOutMax=[]  UintegralTsProdOutMin=[]  UintegralTsProdOutMax=[]  UngainTsProdOutMin=[]  UngainTsProdOutMax=[]  IntegratorContinuousStateAttributes=''  IntegratorStateMustResolveToSignalObject=off  IntegratorRTWStateStorageClass=Auto  FilterContinuousStateAttributes=''  FilterStateMustResolveToSignalObject=off  FilterRTWStateStorageClass=Auto  ParallelPVariant=InternalParameters  IdealPVariant=Disabled  IVariant=InternalParameters  DVariant=Disabled  IntegratorVariant=Continuous  SatVariant=Disabled  AWVariant=Passthrough  PCopyVariant=Disabled  TRVariant=Disabled  FdbkBlocksVariant=Forward  IdealPFdbkVariant=Disabled  SatFdbkVariant=Disabled  DerivativeFilterVariant=Disabled  NVariant=Disabled  NCopyVariant=Disabled_SignalSpec  FilterICVariant=Disabled  IntegratorICVariant=InternalICs  ExternalResetVariant=Disabled  TRSumVariant=Passthrough  SumFdbkVariant=Disabled  SumVariant=Sum_PI  TsampFilterVariant=InternalTs  TsampNgainVariant=Passthrough  TsampIntegralVariant=Passthrough  ExternalSaturationOutDataTypeStr=Inherit: Same as second input
  PWM Generator (DC-DC)1 : spsPWMGeneratorDCDCLib/PWM Generator (DC-DC)  Fsw=5000  Ts=0
  PWM Generator (DC-DC)3 : spsPWMGeneratorDCDCLib/PWM Generator (DC-DC)  Fsw=5000  Ts=0
  Saturation : Saturate
  Saturation1 : Saturate
  Sum : Sum  Inputs=|+-
  Switch : Switch  Criteria=u2 > Threshold
  D_PWM : Outport
  wires:
  MATLAB Function/1(D) -> Saturation/1
  Vpv/1 -> MATLAB Function/1(Vpv)
  Ipv/1 -> MATLAB Function/2(Ipv)
  Saturation1/1 -> PWM Generator (DC-DC)1/1
  V_DC/1 -> Sum/2
  PID Controller/1 -> Saturation1/1
  Sum/1 -> PID Controller/1
  SOC_B/1 -> Compare To Constant/1
  Compare To Constant/1 -> Switch/2
  Saturation/1 -> PWM Generator (DC-DC)3/1
  Switch/1 -> D_PWM/1
  PWM Generator (DC-DC)3/1 -> Switch/3
  PWM Generator (DC-DC)1/1 -> Switch/1
  Constant/1 -> Sum/1

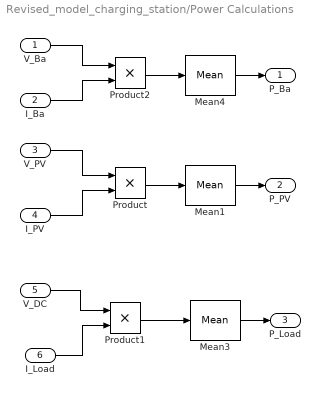
== system Revised_model_charging_station/Power Calculations ==
  V_Ba : Inport
  I_Ba : Inport  Port=2
  V_PV : Inport  Port=3
  I_PV : Inport  Port=4
  V_DC : Inport  Port=5
  I_Load : Inport  Port=6
  Mean1 : spsMeanLib/Mean  Freq=60  Vinit=0  Ts=0
  Mean3 : spsMeanLib/Mean  Freq=60  Vinit=0  Ts=0
  Mean4 : spsMeanLib/Mean  Freq=60  Vinit=0  Ts=0
  Product : Product
  Product1 : Product
  Product2 : Product
  P_Ba : Outport
  P_PV : Outport  Port=2
  P_Load : Outport  Port=3
  wires:
  I_Ba/1 -> Product2/2
  V_Ba/1 -> Product2/1
  V_PV/1 -> Product/1
  I_PV/1 -> Product/2
  V_DC/1 -> Product1/1
  I_Load/1 -> Product1/2
  Mean4/1 -> P_Ba/1
  Product2/1 -> Mean4/1
  Mean1/1 -> P_PV/1
  Product/1 -> Mean1/1
  Mean3/1 -> P_Load/1
  Product1/1 -> Mean3/1

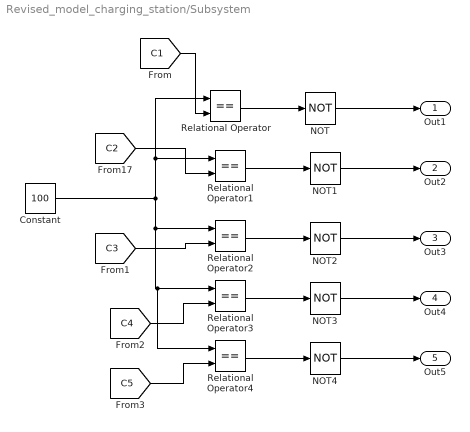
== system Revised_model_charging_station/Subsystem ==
  Constant : Constant  Value=100
  NOT{,1..4} (5 alike) : Logic  Operator=NOT  IconShape=distinctive  AllPortsSameDT=off  OutDataTypeStr=boolean
  Relational Operator{,1..4} (5 alike) : RelationalOperator  Operator===  OutDataTypeStr=boolean  RndMeth=Simplest
  Out1 : Outport
  Out2 : Outport  Port=2
  Out3 : Outport  Port=3
  Out4 : Outport  Port=4
  Out5 : Outport  Port=5
  wires:
  Relational Operator/1 -> NOT/1
  [C1] -> Relational Operator/2
  [C3] -> Relational Operator2/2
  Constant/1 -> Relational Operator1/1, Relational Operator/1, Relational Operator4/1, Relational Operator3/1, Relational Operator2/1
  NOT/1 -> Out1/1
  [C2] -> Relational Operator1/2
  Relational Operator1/1 -> NOT1/1
  Relational Operator2/1 -> NOT2/1
  NOT2/1 -> Out3/1
  Relational Operator3/1 -> NOT3/1
  NOT1/1 -> Out2/1
  NOT3/1 -> Out4/1
  [C4] -> Relational Operator3/2
  [C5] -> Relational Operator4/2
  NOT4/1 -> Out5/1
  Relational Operator4/1 -> NOT4/1

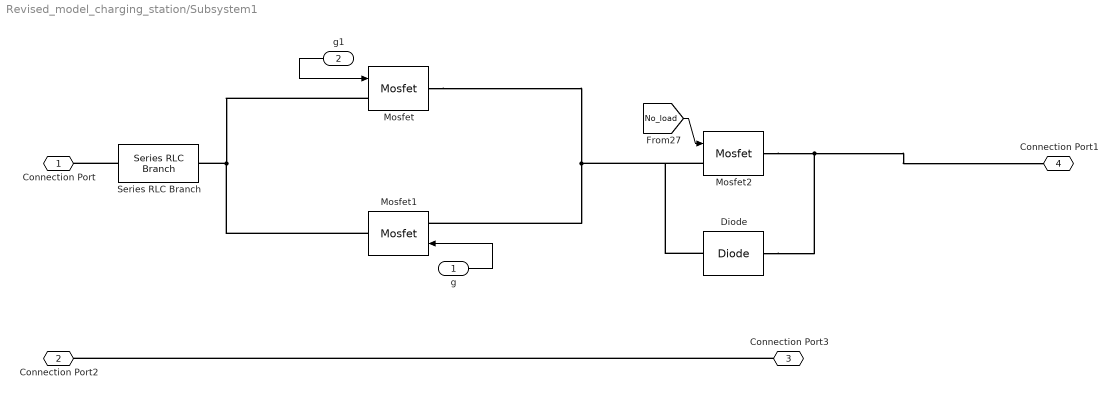
== system Revised_model_charging_station/Subsystem1 ==
  g : Inport
  g1 : Inport  Port=2
  Diode : spsDiodeLib/Diode  Ron=0.001  Lon=0  Vf=0.8  IC=0  UseSnubber=0  Rs=500  Cs=250e-9  Measurements=off
  Mosfet : spsMosfetLib/Mosfet  Ron=0.1  Lon=0  Rd=0.01  Vfd=0  IC=0  Rs=1e5  Cs=inf  Measurements=off
  Mosfet1 : spsMosfetLib/Mosfet  Ron=0.1  Lon=0  Rd=0.01  Vfd=0  IC=0  Rs=1e5  Cs=inf  Measurements=off
  Mosfet2 : spsMosfetLib/Mosfet  Ron=0.1  Lon=0  Rd=0.01  Vfd=0  IC=0  Rs=1e5  Cs=inf  Measurements=off
  Series RLC Branch : spsSeriesRLCBranchLib/Series RLC Branch  LConnTagsString=__new0  RConnTagsString=__new0  BranchType=RL  Resistance=0.05  Inductance=0.3e-3  SetiL0=off  InitialCurrent=0  Capacitance=1e-6  Setx0=off  InitialVoltage=0  Measurements=None
  Connection Port : PMIOPort  Side=Left
  Connection Port2 : PMIOPort  Port=2  Side=Left
  Connection Port3 : PMIOPort  Port=3  Side=Right
  Connection Port1 : PMIOPort  Port=4  Side=Right
  wires:
  g/1 -> Mosfet1/1
  g1/1 -> Mosfet/1
  [No_load] -> Mosfet2/1
  connections:
  Connection Port3/RConn1 -- Connection Port2/RConn1
  Series RLC Branch/LConn1 -- Connection Port/RConn1
  Mosfet/RConn1 -- Diode/RConn1 -- Mosfet2/LConn1 -- Mosfet1/LConn1
  Mosfet1/RConn1 -- Mosfet/LConn1 -- Series RLC Branch/RConn1
  Mosfet2/RConn1 -- Diode/LConn1 -- Connection Port1/RConn1

== system Revised_model_charging_station/Subsystem2 ==
  Constant : Constant  Value=65
  Relational Operator : RelationalOperator  OutDataTypeStr=boolean  RndMeth=Simplest
  Relational Operator1 : RelationalOperator  Operator=<  OutDataTypeStr=boolean  RndMeth=Simplest
  Out1 : Outport
  Out2 : Outport  Port=2
  wires:
  [S_Ba] -> Relational Operator1/1
  [S_Ba] -> Relational Operator/2
  Constant/1 -> Relational Operator/1, Relational Operator1/2
  Relational Operator/1 -> Out1/1
  Relational Operator1/1 -> Out2/1

== system Revised_model_charging_station/Subsystem3 ==
  In1 : Inport
  In2 : Inport  Port=2
  In3 : Inport  Port=3
  In4 : Inport  Port=4
  Add : Sum  Inputs=++++
  Compare To Zero : simulink/Logic and Bit Operations/Compare To Zero  relop===  OutDataTypeStr=boolean
  NOT : Logic  Operator=NOT  IconShape=distinctive  AllPortsSameDT=off  OutDataTypeStr=boolean
  Out1 : Outport
  wires:
  In3/1 -> Add/3
  Add/1 -> Compare To Zero/1
  Compare To Zero/1 -> NOT/1
  In4/1 -> Add/4
  In1/1 -> Add/1
  In2/1 -> Add/2
  NOT/1 -> Out1/1

== matlab function MPPT & GRID CONTROL/MATLAB Function ==
  settings: updateMethod=DISCRETE  sampleTime=1e-4
  data: Vpv input double; D output double; Ipv input double
function D = PandO(Vpv,Ipv)

persistent Dold Pold Vold


if isempty(Dold)
    Dold = 0.35;
    Vold = 17;
    Pold = 120;
end


deltaD = 0.001;

Ppv = Vpv*Ipv;

if (Ppv-Pold) ~= 0
    if (Ppv-Pold) > 0
        if (Vpv-Vold) > 0
            D = Dold - deltaD;
        else
            D = Dold + deltaD;
        end
    else
        if (Vpv-Vold) > 0
            D = Dold + deltaD;
        else
            D = Dold - deltaD;
        end        
    end
else
    D = Dold;
end

Dold = D;
Vold = Vpv;
Pold = Ppv;
